simulink model "InjSys_Co"  (R2016b)
settings: configuration reference "CodeGenConfigSet" (kept outside this file)
values from neighbouring files (symbols this model uses):
  InjSys_ctAirTempSel_C = Calibration.Parameter    [init_InjSys_Co.m]    (also in init_InjSys_Co_SIL.m = Simulink.Parameter)
  InjSys_ctEngTempSel_C = Calibration.Parameter    [init_InjSys_Co.m]    (also in init_InjSys_Co_SIL.m = Simulink.Parameter)
  Rail_ctAirTempSel_C = Calibration.Parameter    [init_InjSys_Co.m]    (also in init_InjSys_Co_SIL.m = Simulink.Parameter)
settings Model: Creator=lenovo  LastModifiedBy=lenovo
settings ConfigSetRef: SourceLocation=Base Workspace

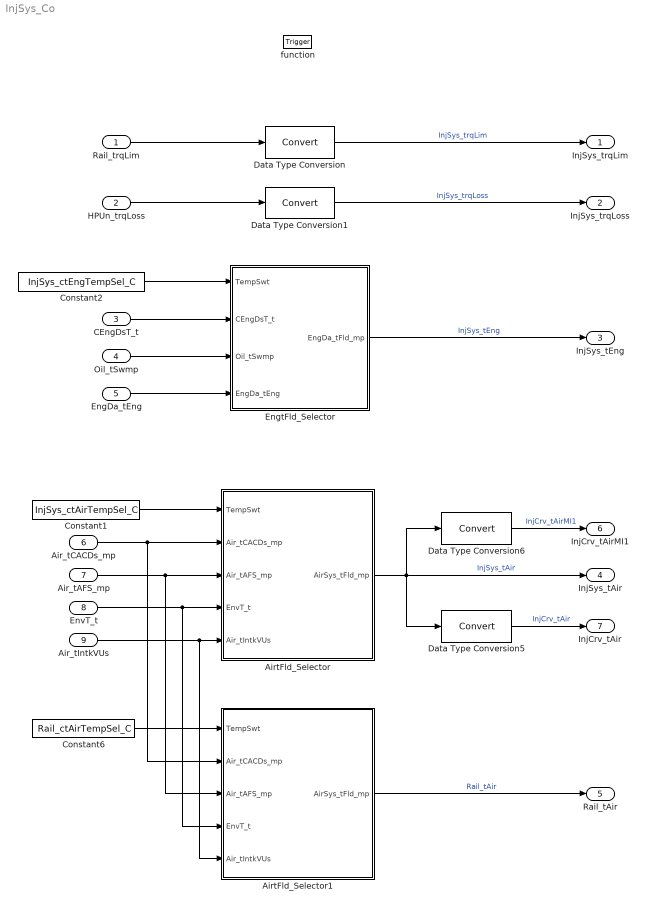
== system InjSys_Co ==
  Rail_trqLim : Inport  Tag=Nm  Description=Torque limitation dependent on fuel temperature  OutMin=0  OutMax=3000  OutDataTypeStr=Trq_Nm
  HPUn_trqLoss : Inport  Tag=Nm  Description=High pressure pump torque demand  Port=2  OutMin=0  OutMax=1000  OutDataTypeStr=Trq_Nm
  CEngDsT_t : Inport  Tag=deg  Description=engine coolant temperature after filter  Port=3  OutMin=-200  OutMax=200  OutDataTypeStr=Temp_deg
  Oil_tSwmp : Inport  Tag=deg  Description=Oil temperature in oil sump  Port=4  OutMin=-50  OutMax=200  OutDataTypeStr=Temp_deg
  EngDa_tEng : Inport  Tag=deg  Description=Engine temperature  Port=5  OutMin=-1000  OutMax=1000  OutDataTypeStr=Temp_deg
  Air_tCACDs_mp : Inport  Tag=deg  Description=Charge-air temperature downstream from charge-air cooler  Port=6  OutMin=-200  OutMax=200  OutDataTypeStr=Temp_deg
  Air_tAFS_mp : Inport  Tag=deg  Description=Induction air temperature at the HFM  Port=7  OutMin=-200  OutMax=200  OutDataTypeStr=Temp_deg
  EnvT_t : Inport  Tag=deg  Description=Environmental temperature  Port=8  OutMin=-200  OutMax=200  OutDataTypeStr=Temp_deg
  Air_tIntkVUs : Inport  Tag=deg  Description=Intake air temperature upstream of the inlet valve  Port=9  OutMin=-200  OutMax=200  OutDataTypeStr=Temp_deg
  function : TriggerPort  TriggerType=function-call  VariantControl=Variant
  AirtFld_Selector : Subsystem
  AirtFld_Selector1 : Subsystem
  Constant1 : Constant  Value=InjSys_ctAirTempSel_C
  Constant2 : Constant  Value=InjSys_ctEngTempSel_C
  Constant6 : Constant  Value=Rail_ctAirTempSel_C
  Data Type Conversion{,1,5..6} (4 alike) : DataTypeConversion
  EngtFld_Selector : Subsystem
  InjSys_trqLim : Outport  Tag=Nm  Description=Torque limitation of injection system  OutMin=-3276.8  OutMax=3276.7  OutDataTypeStr=Trq_Nm
  InjSys_trqLoss : Outport  Tag=Nm  Description=Torque loss of injection system  Port=2  OutMin=-3276.8  OutMax=3276.7  OutDataTypeStr=Trq_Nm
  InjSys_tEng : Outport  Tag=deg  Description=Engine temperature selected for the injection system  Port=3  OutMin=-1000  OutMax=1000  OutDataTypeStr=Temp_deg
  InjSys_tAir : Outport  Tag=deg  Description=Intake air temperature selected for the injection system  Port=4  OutMin=-1000  OutMax=1000  OutDataTypeStr=Temp_deg
  Rail_tAir : Outport  Tag=deg  Description=Intake air temperature for the Rail subsystem  Port=5  OutMin=-1000  OutMax=1000  OutDataTypeStr=Temp_deg
  InjCrv_tAirMI1 : Outport  Tag=deg  Description=Chosen temperature from the temperature field on the induction system  Port=6  OutMin=-50  OutMax=150  OutDataTypeStr=Temp_deg
  InjCrv_tAir : Outport  Tag=deg  Description=Air temperature for environment corrections  Port=7  OutMin=-50  OutMax=150  OutDataTypeStr=Temp_deg
  wires:
  Data Type Conversion/1 -> InjSys_trqLim/1  "InjSys_trqLim"
  Data Type Conversion1/1 -> InjSys_trqLoss/1  "InjSys_trqLoss"
  HPUn_trqLoss/1 -> Data Type Conversion1/1
  Rail_trqLim/1 -> Data Type Conversion/1
  AirtFld_Selector/1(AirSys_tFld_mp) -> Data Type Conversion5/1, InjSys_tAir/1, Data Type Conversion6/1  "InjSys_tAir"
  EngtFld_Selector/1(EngDa_tFld_mp) -> InjSys_tEng/1  "InjSys_tEng"
  AirtFld_Selector1/1(AirSys_tFld_mp) -> Rail_tAir/1  "Rail_tAir"
  Data Type Conversion5/1 -> InjCrv_tAir/1  "InjCrv_tAir"
  Data Type Conversion6/1 -> InjCrv_tAirMI1/1  "InjCrv_tAirMI1"
  Constant2/1 -> EngtFld_Selector/1(TempSwt)
  CEngDsT_t/1 -> EngtFld_Selector/2(CEngDsT_t)
  Oil_tSwmp/1 -> EngtFld_Selector/3(Oil_tSwmp)
  EngDa_tEng/1 -> EngtFld_Selector/4(EngDa_tEng)
  Constant1/1 -> AirtFld_Selector/1(TempSwt)
  Air_tCACDs_mp/1 -> AirtFld_Selector/2(Air_tCACDs_mp), AirtFld_Selector1/2(Air_tCACDs_mp)
  Air_tAFS_mp/1 -> AirtFld_Selector/3(Air_tAFS_mp), AirtFld_Selector1/3(Air_tAFS_mp)
  EnvT_t/1 -> AirtFld_Selector1/4(EnvT_t), AirtFld_Selector/4(EnvT_t)
  Air_tIntkVUs/1 -> AirtFld_Selector1/5(Air_tIntkVUs), AirtFld_Selector/5(Air_tIntkVUs)
  Constant6/1 -> AirtFld_Selector1/1(TempSwt)

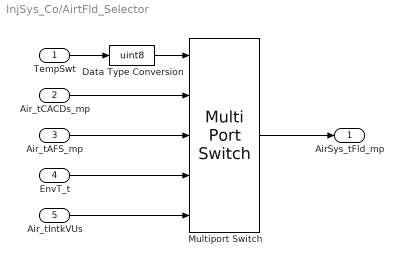
== system InjSys_Co/AirtFld_Selector ==
  TempSwt : Inport
  Air_tCACDs_mp : Inport  Tag=deg  Description=Charge-air temperature downstream from charge-air cooler  Port=2
  Air_tAFS_mp : Inport  Tag=deg  Description=Induction air temperature at the HFM  Port=3
  EnvT_t : Inport  Tag=deg  Description=Environmental temperature  Port=4
  Air_tIntkVUs : Inport  Tag=deg  Description=Intake air temperature upstream of the inlet valve  Port=5
  Data Type Conversion : DataTypeConversion  OutDataTypeStr=uint8
  Multiport Switch : MultiPortSwitch  DataPortOrder=Zero-based contiguous  Inputs=4
  AirSys_tFld_mp : Outport  Tag=deg  Description=Engine temperature field
  wires:
  Air_tCACDs_mp/1 -> Multiport Switch/2
  Multiport Switch/1 -> AirSys_tFld_mp/1
  EnvT_t/1 -> Multiport Switch/4
  Air_tAFS_mp/1 -> Multiport Switch/3
  Data Type Conversion/1 -> Multiport Switch/1
  TempSwt/1 -> Data Type Conversion/1
  Air_tIntkVUs/1 -> Multiport Switch/5

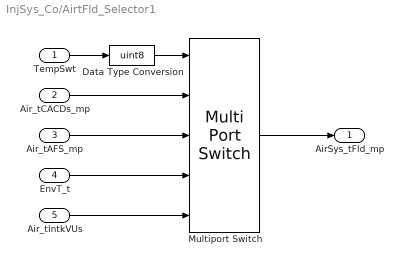
== system InjSys_Co/AirtFld_Selector1 ==
  TempSwt : Inport
  Air_tCACDs_mp : Inport  Tag=deg  Description=Charge-air temperature downstream from charge-air cooler  Port=2
  Air_tAFS_mp : Inport  Tag=deg  Description=Induction air temperature at the HFM  Port=3
  EnvT_t : Inport  Tag=deg  Description=Environmental temperature  Port=4
  Air_tIntkVUs : Inport  Tag=deg  Description=Intake air temperature upstream of the inlet valve  Port=5
  Data Type Conversion : DataTypeConversion  OutDataTypeStr=uint8
  Multiport Switch : MultiPortSwitch  DataPortOrder=Zero-based contiguous  Inputs=4
  AirSys_tFld_mp : Outport  Tag=deg  Description=Engine temperature field
  wires:
  Air_tCACDs_mp/1 -> Multiport Switch/2
  Multiport Switch/1 -> AirSys_tFld_mp/1
  EnvT_t/1 -> Multiport Switch/4
  Air_tAFS_mp/1 -> Multiport Switch/3
  Data Type Conversion/1 -> Multiport Switch/1
  TempSwt/1 -> Data Type Conversion/1
  Air_tIntkVUs/1 -> Multiport Switch/5

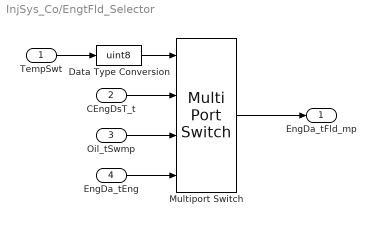
== system InjSys_Co/EngtFld_Selector ==
  TempSwt : Inport
  CEngDsT_t : Inport  Tag=deg  Description=engine coolant temperature after filter  Port=2
  Oil_tSwmp : Inport  Tag=deg  Description=Oil temperature in oil sump  Port=3
  EngDa_tEng : Inport  Tag=deg  Description=Engine temperature  Port=4
  Data Type Conversion : DataTypeConversion  OutDataTypeStr=uint8
  Multiport Switch : MultiPortSwitch  DataPortOrder=Zero-based contiguous
  EngDa_tFld_mp : Outport  Tag=deg  Description=Engine temperature field
  wires:
  CEngDsT_t/1 -> Multiport Switch/2
  Multiport Switch/1 -> EngDa_tFld_mp/1
  EngDa_tEng/1 -> Multiport Switch/4
  Oil_tSwmp/1 -> Multiport Switch/3
  Data Type Conversion/1 -> Multiport Switch/1
  TempSwt/1 -> Data Type Conversion/1
